simulink model "slprimes"  (Simulink 6.0)
settings: Solver=FixedStepDiscrete  StartTime=0  StopTime=inf  FixedStep=1  RelTol=1e-3
StopFcn:
  | try, fprintf('Simulation: sprime3\nPrime numbers from 2:%d : \n',n);disp(p); end
undefined symbols (not defined in the file or in its folder): gcbh, n
libraries: lights x3
settings Model: Tag=MergeExample  Creator=The MathWorks Inc.  LastModifiedBy=batserve  ExtModeTrigMode=oneshot  ExtModeArmWhenConnect=off  ExtModeAutoUpdateStatusClock=off
settings DataIOCC: MaxDataPoints=1  SaveFormat=Structure  SaveOutput=off  SaveTime=off  SignalLoggingName=logsOut
settings OptimizationCC: BlockReduction=off
settings DebuggingCC: CheckExecutionContextPreStartOutputMsg=on  CheckExecutionContextRuntimeOutputMsg=on  SolverPrmCheckMsg=none  UnnecessaryDatatypeConvMsg=warning
settings HardwareCC: TargetUnknown=on
settings RTWCC: GenCodeOnly=on

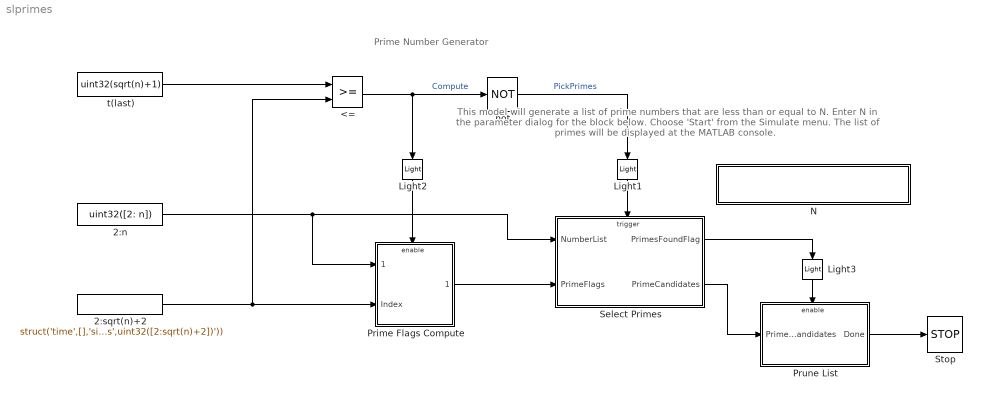
== system slprimes ==
  note: This model will generate a list of prime numbers that
      | are less than or equal to N.  Enter N in the parameter
      | dialog for the block below.  Choose 'Start' from the
      | Simulate menu.  The list of primes will be displayed
      | at the MATLAB console.
  note: Prime Number Generator
  " <=" : RelationalOperator  InputSameDT=on
  2:n : Constant  Value=uint32([2: n])
  2:sqrt(n)+2 : FromWorkspace  VariableName=struct('time',[],'signals',struct('values',uint32([2:sqrt(n)+2])'))  SampleTime=1  Interpolate=off  OutputAfterFinalValue=Holding final value
  Light1 : lights/Light  Orientation=down  state=Stop
  Light2 : lights/Light  Orientation=down  state=Stop
  Light3 : lights/Light  Orientation=down  state=Stop
  N : Subsystem  InitFcn=assignin('base','n',evalin('base',get_param(gcbh,'N')));  PropExecContextAcrossSSBoundary=on  mask(Primes Input){N=25}
      mask prompts: N "Primes up to:"
      mask Display: disp(N)
  Prime Flags Compute : Subsystem  TreatAsAtomicUnit=on  PropExecContextAcrossSSBoundary=on
  Prune List : Subsystem  TreatAsAtomicUnit=on  PropExecContextAcrossSSBoundary=on
  Select Primes : Subsystem  TreatAsAtomicUnit=on  PropExecContextAcrossSSBoundary=on
  Stop : Stop
  not : Logic  Operator=NOT  Inputs=1
  t(last) : Constant  Value=uint32(sqrt(n)+1)
  wires:
  " <="/1 -> not/1, Light2/1  "Compute"
  Prime Flags Compute/1(PrimeFlags) -> Select Primes/2(PrimeFlags)
  Select Primes/2(PrimeCandidates) -> Prune List/1(PrimeCandidates)
  Light1/1 -> Select Primes/Trigger
  Light2/1 -> Prime Flags Compute/Enable
  Light3/1 -> Prune List/Enable
  not/1 -> Light1/1  "PickPrimes"
  Prune List/1(Done) -> Stop/1
  Select Primes/1(PrimesFoundFlag) -> Light3/1
  2:n/1 -> Select Primes/1(NumberList), Prime Flags Compute/1(NumberList)
  2:sqrt(n)+2/1 -> Prime Flags Compute/2(Index), " <="/2
  t(last)/1 -> " <="/1

== system slprimes/N ==

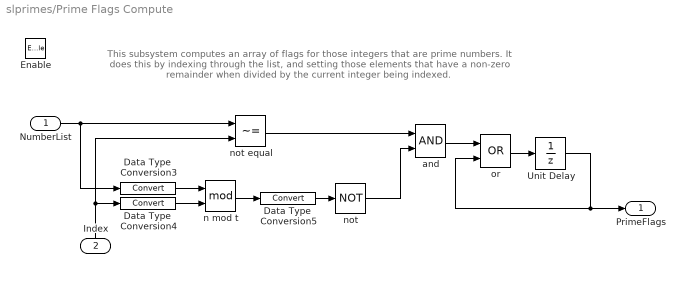
== system slprimes/Prime Flags Compute ==
  note: This subsystem computes an array of flags for those integers
      | that are prime numbers.  It does this by indexing through the
      | list, and setting those elements that have a non-zero remainder
      | when divided by the current integer being indexed.
  NumberList : Inport  Port=1  LatchInput=off
  Index : Inport  Orientation=up  Port=2  LatchInput=off
  Enable : EnablePort
  Data Type  Conversion3 : DataTypeConversion  OutDataTypeMode=double  SaturateOnIntegerOverflow=on  RndMeth=Zero
  Data Type  Conversion4 : DataTypeConversion  OutDataTypeMode=double  SaturateOnIntegerOverflow=on  RndMeth=Zero
  Data Type  Conversion5 : DataTypeConversion  OutDataTypeMode=boolean  SaturateOnIntegerOverflow=on  RndMeth=Zero
  Unit Delay : UnitDelay
  and : Logic
  n mod t : Math  Operator=mod  SaturateOnIntegerOverflow=on
  not : Logic  Operator=NOT  Inputs=1
  not equal : RelationalOperator  Operator=~=  InputSameDT=on
  or : Logic  Operator=OR
  PrimeFlags : Outport  InitialOutput=0
  wires:
  NumberList/1 -> not equal/1, Data Type  Conversion3/1
  Data Type  Conversion3/1 -> n mod t/1
  Data Type  Conversion4/1 -> n mod t/2
  not equal/1 -> and/1
  Unit Delay/1 -> PrimeFlags/1, or/2
  and/1 -> or/1
  not/1 -> and/2
  or/1 -> Unit Delay/1
  n mod t/1 -> Data Type  Conversion5/1
  Data Type  Conversion5/1 -> not/1
  Index/1 -> not equal/2, Data Type  Conversion4/1

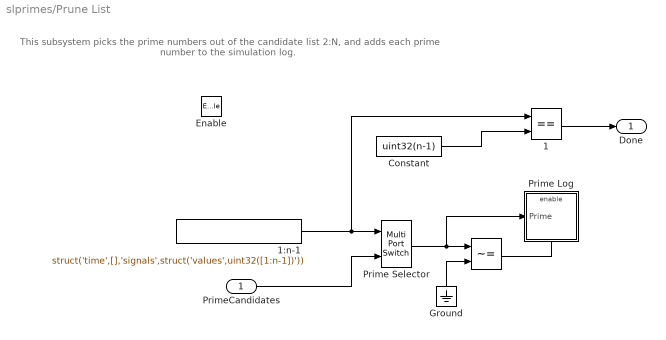
== system slprimes/Prune List ==
  note: This subsystem picks the prime numbers out of the candidate list
      | 2:N, and adds each prime number to the simulation log.
  PrimeCandidates : Inport  Port=1  LatchInput=off
  Enable : EnablePort
  " " : RelationalOperator  Operator=~=  InputSameDT=on
  " 1" : RelationalOperator  Operator===  InputSameDT=on
  1:n-1 : FromWorkspace  VariableName=struct('time',[],'signals',struct('values',uint32([1:n-1])'))  SampleTime=1  Interpolate=off  OutputAfterFinalValue=Holding final value
  Constant : Constant  Value=uint32(n-1)
  Ground : Ground  Orientation=up
  Prime Selector : MultiPortSwitch  Inputs=1  SaturateOnIntegerOverflow=on  InputSameDT=on
  Prime Log : Subsystem  TreatAsAtomicUnit=on  PropExecContextAcrossSSBoundary=on
  Done : Outport
  wires:
  Constant/1 -> " 1"/2
  " 1"/1 -> Done/1
  PrimeCandidates/1 -> Prime Selector/2
  Ground/1 -> " "/2
  " "/1 -> Prime Log/Enable
  Prime Selector/1 -> " "/1, Prime Log/1(Prime)
  1:n-1/1 -> Prime Selector/1, " 1"/1

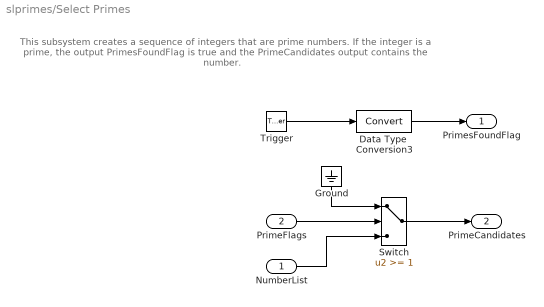
== system slprimes/Select Primes ==
  note: This subsystem creates a sequence of integers that are prime
      | numbers.  If the integer is a prime, the output PrimesFoundFlag
      | is true and the PrimeCandidates output contains the number.
  NumberList : Inport  Port=1  LatchInput=off
  PrimeFlags : Inport  Port=2  LatchInput=off
  Trigger : TriggerPort  ShowOutputPort=on  OutputDataType=int8
  Data Type  Conversion3 : DataTypeConversion  OutDataTypeMode=boolean  SaturateOnIntegerOverflow=on  RndMeth=Zero
  Ground : Ground  Orientation=down
  Switch : Switch  Threshold=1  SaturateOnIntegerOverflow=on  InputSameDT=on
  PrimesFoundFlag : Outport
  PrimeCandidates : Outport  Port=2
  wires:
  PrimeFlags/1 -> Switch/2
  NumberList/1 -> Switch/3
  Switch/1 -> PrimeCandidates/1
  Ground/1 -> Switch/1
  Trigger/1 -> Data Type  Conversion3/1
  Data Type  Conversion3/1 -> PrimesFoundFlag/1

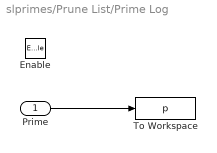
== system slprimes/Prune List/Prime Log ==
  Prime : Inport  Port=1  LatchInput=off
  Enable : EnablePort
  To Workspace : ToWorkspace  VariableName=p  SampleTime=-1  SaveFormat=Array
  wires:
  Prime/1 -> To Workspace/1
